simulink model "SistemaP3"  (R2024b)
settings: Solver=ode15s  StartTime=0.0  StopTime=10.0  MaxStep=1e-3  RelTol=1e-3
settings Model: Creator=HP  LastModifiedBy=DELL
settings SolverCC: AlgebraicLoopSolver=TrustRegion
settings DataIOCC: ReturnWorkspaceOutputs=off  TimeSaveName=t
settings DebuggingCC: AlgebraicLoopMsg=none  ArtificialAlgebraicLoopMsg=none  MaxConsecutiveZCsMsg=none  InheritedTsInSrcMsg=none  UnconnectedInputMsg=warning  UnconnectedOutputMsg=warning  UnconnectedLineMsg=warning  UnknownTsInhSupMsg=none  OperatingPointInterfaceChecksumMismatchMsg=none
settings ModelReferenceCC: EnableRefExpFcnMdlSchedulingChecks=on
settings RTWCC: GPUComputeCapability=3.5  DLArmComputeVersion=19.05

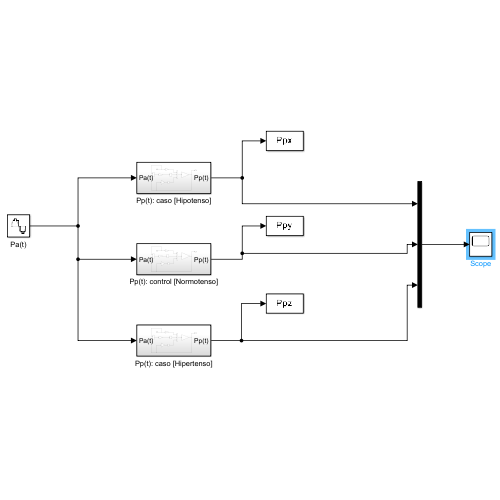
[thumbnail: Simulink's stored preview of the top-level diagram]
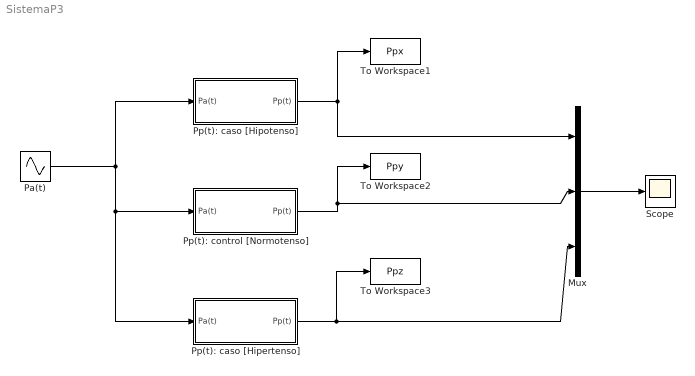
== system SistemaP3 ==
  Mux : Mux  Inputs=3
  Pa(t) : Sin  Bias=0.8  Frequency=2*pi*95/60  SampleTime=0.001
  Pp(t): caso [Hipertenso] : Subsystem
  Pp(t): caso [Hipotenso] : Subsystem
  Pp(t): control [Normotenso] : Subsystem
  Scope : Scope
  To Workspace1 : ToWorkspace  VariableName=Ppx  SampleTime=-1
  To Workspace2 : ToWorkspace  VariableName=Ppy  SampleTime=-1
  To Workspace3 : ToWorkspace  VariableName=Ppz  SampleTime=-1
  wires:
  Pa(t)/1 -> Pp(t): caso [Hipertenso]/1(Pa(t)), Pp(t): control [Normotenso]/1(Pa(t)), Pp(t): caso [Hipotenso]/1(Pa(t))
  Pp(t): caso [Hipotenso]/1(Pp(t)) -> To Workspace1/1, Mux/1
  Pp(t): control [Normotenso]/1(Pp(t)) -> To Workspace2/1, Mux/2
  Pp(t): caso [Hipertenso]/1(Pp(t)) -> To Workspace3/1, Mux/3
  Mux/1 -> Scope/1

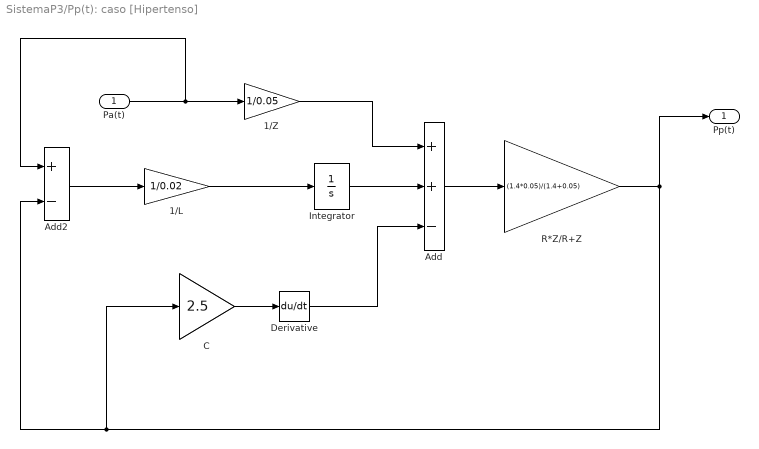
== system SistemaP3/Pp(t): caso [Hipertenso] ==
  Pa(t) : Inport
  1/L : Gain  Gain=1/0.02
  1/Z : Gain  Gain=1/0.05
  Add : Sum  Inputs=++-
  Add2 : Sum  Inputs=+-
  C : Gain  Gain=2.5
  Derivative : Derivative
  Integrator : Integrator
  R*Z/R+Z : Gain  Gain=(1.4*0.05)/(1.4+0.05)
  Pp(t) : Outport  VectorParamsAs1DForOutWhenUnconnected=off
  wires:
  Add/1 -> R*Z/R+Z/1
  Add2/1 -> 1/L/1
  C/1 -> Derivative/1
  Derivative/1 -> Add/3
  Integrator/1 -> Add/2
  1/L/1 -> Integrator/1
  1/Z/1 -> Add/1
  Pa(t)/1 -> Add2/1, 1/Z/1
  R*Z/R+Z/1 -> Pp(t)/1, Add2/2, C/1

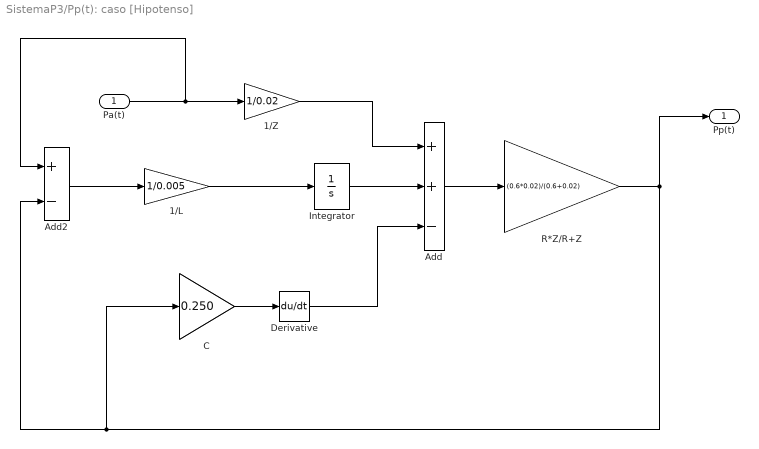
== system SistemaP3/Pp(t): caso [Hipotenso] ==
  Pa(t) : Inport
  1/L : Gain  Gain=1/0.005
  1/Z : Gain  Gain=1/0.02
  Add : Sum  Inputs=++-
  Add2 : Sum  Inputs=+-
  C : Gain  Gain=0.250
  Derivative : Derivative
  Integrator : Integrator
  R*Z/R+Z : Gain  Gain=(0.6*0.02)/(0.6+0.02)
  Pp(t) : Outport  VectorParamsAs1DForOutWhenUnconnected=off
  wires:
  Add/1 -> R*Z/R+Z/1
  Add2/1 -> 1/L/1
  C/1 -> Derivative/1
  Derivative/1 -> Add/3
  Integrator/1 -> Add/2
  1/L/1 -> Integrator/1
  1/Z/1 -> Add/1
  Pa(t)/1 -> Add2/1, 1/Z/1
  R*Z/R+Z/1 -> Pp(t)/1, Add2/2, C/1

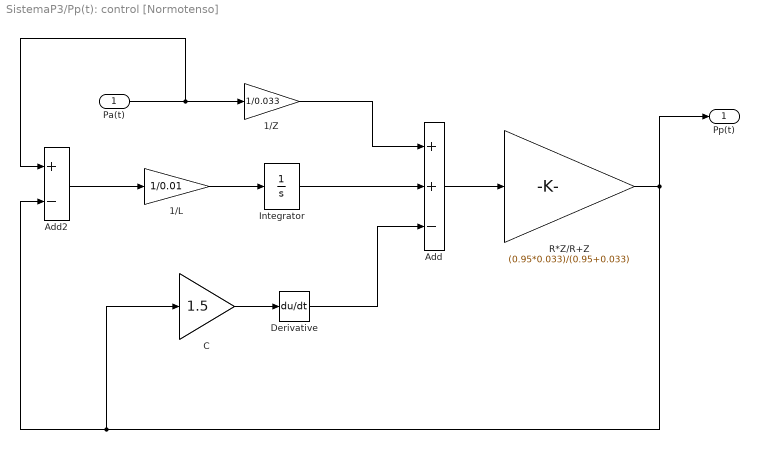
== system SistemaP3/Pp(t): control [Normotenso] ==
  Pa(t) : Inport
  1/L : Gain  Gain=1/0.01
  1/Z : Gain  Gain=1/0.033
  Add : Sum  Inputs=++-
  Add2 : Sum  Inputs=+-
  C : Gain  Gain=1.5
  Derivative : Derivative
  Integrator : Integrator
  R*Z/R+Z : Gain  Gain=(0.95*0.033)/(0.95+0.033)
  Pp(t) : Outport  VectorParamsAs1DForOutWhenUnconnected=off
  wires:
  Add/1 -> R*Z/R+Z/1
  Add2/1 -> 1/L/1
  C/1 -> Derivative/1
  Derivative/1 -> Add/3
  Integrator/1 -> Add/2
  1/L/1 -> Integrator/1
  1/Z/1 -> Add/1
  Pa(t)/1 -> Add2/1, 1/Z/1
  R*Z/R+Z/1 -> Pp(t)/1, Add2/2, C/1
